simulink model "SWC_TCF"  (R2020a)
settings: Solver=FixedStepDiscrete  StartTime=0.0  StopTime=0.01  FixedStep=0.001  RelTol=1e-3
values from neighbouring files (symbols this model uses):
  CAL_TCF_AgTrqTubeCAy_af32 = 0.0    [SWC_TCF_DataDictionary.sldd]
  CAL_TCF_flgUsePlossCompa_b = 0.0    [SWC_TCF_DataDictionary.sldd]
  CAL_TCF_HiSpdDirStop_f32 = 0.0    [SWC_TCF_DataDictionary.sldd]
  CAL_TCF_HiTrqDirStop_f32 = 0.0    [SWC_TCF_DataDictionary.sldd]
  CAL_TCF_IsCutOffFrq_f32 = 0.0    [SWC_TCF_DataDictionary.sldd]
  CAL_TCF_IsPwrLosCAx_af32 = 0.0    [SWC_TCF_DataDictionary.sldd]
  CAL_TCF_LdSubLqCAzGen_af32 = 0.0    [SWC_TCF_DataDictionary.sldd]
  CAL_TCF_LdSubLqCAzMot_af32 = 0.0    [SWC_TCF_DataDictionary.sldd]
  CAL_TCF_LdSubLqIdCAx_af32 = 0.0    [SWC_TCF_DataDictionary.sldd]
  CAL_TCF_LdSubLqIqCAy_af32 = 0.0    [SWC_TCF_DataDictionary.sldd]
  CAL_TCF_LoSpdDirStop_f32 = 0.0    [SWC_TCF_DataDictionary.sldd]
  CAL_TCF_LoTrqDirStop_f32 = 0.0    [SWC_TCF_DataDictionary.sldd]
  CAL_TCF_MotorPole_u8 = 0.0    [SWC_TCF_DataDictionary.sldd]
  CAL_TCF_NPwrLosCAy_af32 = 0.0    [SWC_TCF_DataDictionary.sldd]
  CAL_TCF_Psi_f32 = 0.0    [SWC_TCF_DataDictionary.sldd]
  CAL_TCF_PwrCompaElectCAz_af32 = 0.0    [SWC_TCF_DataDictionary.sldd]
  CAL_TCF_PwrCompaIsCAy_af32 = 0.0    [SWC_TCF_DataDictionary.sldd]
  CAL_TCF_PwrCompaSpdCAx_af32 = 0.0    [SWC_TCF_DataDictionary.sldd]
  CAL_TCF_PwrInputCutOffFrq_f32 = 0.0    [SWC_TCF_DataDictionary.sldd]
  CAL_TCF_PwrLossCAz_af32 = 0.0    [SWC_TCF_DataDictionary.sldd]
  CAL_TCF_PwrTrqCalcSpdThrH_f32 = 0.0    [SWC_TCF_DataDictionary.sldd]
  CAL_TCF_PwrTrqCalcSpdThrL_f32 = 0.0    [SWC_TCF_DataDictionary.sldd]
  CAL_TCF_PwrTrqTubeCAy_af32 = 0.0    [SWC_TCF_DataDictionary.sldd]
  CAL_TCF_SpeedCtlMode_u8 = 0.0    [SWC_TCF_DataDictionary.sldd]
  CAL_TCF_TempStrMax_f32 = 0.0    [SWC_TCF_DataDictionary.sldd]
  CAL_TCF_TempStrMin_f32 = 0.0    [SWC_TCF_DataDictionary.sldd]
  CAL_TCF_TempStrPlossFact_f32 = 0.0    [SWC_TCF_DataDictionary.sldd]
  CAL_TCF_TrqCalcMonCountTrh_s16 = 0.0    [SWC_TCF_DataDictionary.sldd]
  CAL_TCF_TrqCalcMonDebTrh_s16 = 0.0    [SWC_TCF_DataDictionary.sldd]
  CAL_TCF_TrqCalcMonErrRst_b = 0.0    [SWC_TCF_DataDictionary.sldd]
  CAL_TCF_TrqMechCutOffFrq_f32 = 0.0    [SWC_TCF_DataDictionary.sldd]
  CAL_TCF_TrqTubeNCAx_af32 = 0.0    [SWC_TCF_DataDictionary.sldd]
  GLB_TCF_BwELect_u8 = 0.0    [SWC_TCF_DataDictionary.sldd]
  GLB_TCF_BwGene_u8 = 0.0    [SWC_TCF_DataDictionary.sldd]
  GLB_TCF_CircAge_f32 = 0.0    [SWC_TCF_DataDictionary.sldd]
  GLB_TCF_DigtValue_u16 = 0.0    [SWC_TCF_DataDictionary.sldd]
  GLB_TCF_FwELect_u8 = 0.0    [SWC_TCF_DataDictionary.sldd]
  GLB_TCF_FwGene_u8 = 0.0    [SWC_TCF_DataDictionary.sldd]
  GLB_TCF_MotorBw_u8 = 0.0    [SWC_TCF_DataDictionary.sldd]
  GLB_TCF_MotorFw_u8 = 0.0    [SWC_TCF_DataDictionary.sldd]
  GLB_TCF_MotorStop_u8 = 0.0    [SWC_TCF_DataDictionary.sldd]
  GLB_TCF_NegvTrq_u8 = 0.0    [SWC_TCF_DataDictionary.sldd]
  GLB_TCF_PosvTrq_u8 = 0.0    [SWC_TCF_DataDictionary.sldd]
  GLB_TCF_ZeroTrq_u8 = 0.0    [SWC_TCF_DataDictionary.sldd]
  PRV_CalFltFrq_1ms = 0.0    [SWC_TCF_DataDictionary.sldd]
  PRV_IsCalFltFrq_1ms = 0.0    [SWC_TCF_DataDictionary.sldd]
  Tbl_cos_table = 0.0    [SWC_TCF_DataDictionary.sldd]
  Tbl_sin_table = 0.0    [SWC_TCF_DataDictionary.sldd]
  TCF_PwrCompaGenCAz_af32 = 0.0    [SWC_TCF_DataDictionary.sldd]
undefined symbols (not defined in the file or in its folder): CAL_TOM_AgTrqFltTs_f32, CAL_TOM_PwrTrqFltTs_f32
libraries: simulink x9
(part 1 of 2)
settings Model: DataDictionary=SWC_TCF_DataDictionary.sldd  EnableAccessToBaseWorkspace=off  Creator=dongliyuan  LastModifiedBy=zhangjunren
settings DataIOCC: SaveFormat=StructureWithTime
settings OptimizationCC: DefaultParameterBehavior=Inlined  DefaultUnderspecifiedDataType=single  EnhancedBackFolding=on  PassReuseOutputArgsAs=Individual arguments  ZeroExternalMemoryAtStartup=off  ZeroInternalMemoryAtStartup=off  OptimizeBlockOrder=speed  DifferentSizesBufferReuse=on  OptimizationCustomize=off  EfficientTunableParamExpr=on
settings DebuggingCC: SignalInfNanChecking=warning  ParameterPrecisionLossMsg=none  ParameterTunabilityLossMsg=error  UnnecessaryDatatypeConvMsg=warning  VectorMatrixConversionMsg=warning  StrictBusMsg=WarnOnBusTreatedAsVector  NonBusSignalsTreatedAsBus=warning
settings ModelReferenceCC: ModelReferenceNumInstancesAllowed=Single
settings SFSimCC: MATLABDynamicMemAlloc=off
settings RTWCC: SystemTargetFile=ert.tlc  GenCodeOnly=on  TemplateMakefile=ert_default_tmf
settings RTWCC: CustomSourceCode=|
  | #include "set_get_data.h"
  | #include "L2Sample_FS.h"
settings CodeAppCC: ForceParamTrailComments=on  IgnoreCustomStorageClasses=off  OperatorAnnotations=on  SimulinkDataObjDesc=on  SFDataObjDesc=on  InsertBlockDesc=on
settings ERTTargetCC: TargetLangStandard=C99 (ISO)  UtilityFuncGeneration=Shared location  IncludeMdlTerminateFcn=off  SupportNonFinite=off  SupportComplex=off  GenerateASAP2=on  InlinedParameterPlacement=NonHierarchical  ERTCustomFileTemplate=example_file_process.tlc  EnableUserReplacementTypes=on

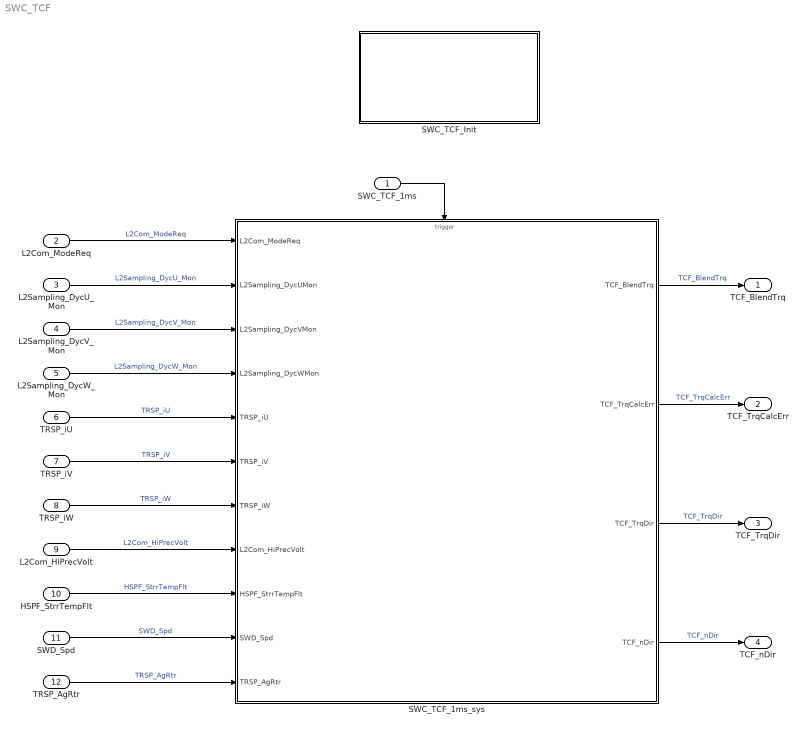
== system SWC_TCF ==
  SWC_TCF_1ms : Inport  SampleTime=0.001  OutputFunctionCall=on
  L2Com_ModeReq : Inport  Port=2  OutDataTypeStr=uint8  PortDimensions=1
  L2Sampling_DycU_Mon : Inport  Port=3  OutDataTypeStr=single  PortDimensions=1
  L2Sampling_DycV_Mon : Inport  Port=4  OutDataTypeStr=single  PortDimensions=1
  L2Sampling_DycW_Mon : Inport  Port=5  OutDataTypeStr=single  PortDimensions=1
  TRSP_iU : Inport  Port=6  OutDataTypeStr=single  PortDimensions=1
  TRSP_iV : Inport  Port=7  OutDataTypeStr=single  PortDimensions=1
  TRSP_iW : Inport  Port=8  OutDataTypeStr=single  PortDimensions=1
  L2Com_HiPrecVolt : Inport  Port=9  OutDataTypeStr=single  PortDimensions=1
  HSPF_StrrTempFlt : Inport  Port=10
  SWD_Spd : Inport  Port=11
  TRSP_AgRtr : Inport  Port=12
  SWC_TCF_1ms_sys : Subsystem
  SWC_TCF_Init : Subsystem
  TCF_BlendTrq : Outport
  TCF_TrqCalcErr : Outport  Port=2
  TCF_TrqDir : Outport  Port=3
  TCF_nDir : Outport  Port=4
  wires:
  L2Sampling_DycU_Mon/1 -> SWC_TCF_1ms_sys/2(L2Sampling_DycUMon)  "L2Sampling_DycU_Mon"
  L2Sampling_DycV_Mon/1 -> SWC_TCF_1ms_sys/3(L2Sampling_DycVMon)  "L2Sampling_DycV_Mon"
  L2Sampling_DycW_Mon/1 -> SWC_TCF_1ms_sys/4(L2Sampling_DycWMon)  "L2Sampling_DycW_Mon"
  L2Com_HiPrecVolt/1 -> SWC_TCF_1ms_sys/8(L2Com_HiPrecVolt)  "L2Com_HiPrecVolt"
  L2Com_ModeReq/1 -> SWC_TCF_1ms_sys/1(L2Com_ModeReq)  "L2Com_ModeReq"
  SWC_TCF_1ms/1 -> SWC_TCF_1ms_sys/Trigger
  HSPF_StrrTempFlt/1 -> SWC_TCF_1ms_sys/9(HSPF_StrrTempFlt)  "HSPF_StrrTempFlt"
  SWD_Spd/1 -> SWC_TCF_1ms_sys/10(SWD_Spd)  "SWD_Spd"
  TRSP_AgRtr/1 -> SWC_TCF_1ms_sys/11(TRSP_AgRtr)  "TRSP_AgRtr"
  TRSP_iU/1 -> SWC_TCF_1ms_sys/5(TRSP_iU)  "TRSP_iU"
  TRSP_iV/1 -> SWC_TCF_1ms_sys/6(TRSP_iV)  "TRSP_iV"
  TRSP_iW/1 -> SWC_TCF_1ms_sys/7(TRSP_iW)  "TRSP_iW"
  SWC_TCF_1ms_sys/1(TCF_BlendTrq) -> TCF_BlendTrq/1  "TCF_BlendTrq"
  SWC_TCF_1ms_sys/2(TCF_TrqCalcErr) -> TCF_TrqCalcErr/1  "TCF_TrqCalcErr"
  SWC_TCF_1ms_sys/3(TCF_TrqDir) -> TCF_TrqDir/1  "TCF_TrqDir"
  SWC_TCF_1ms_sys/4(TCF_nDir) -> TCF_nDir/1  "TCF_nDir"

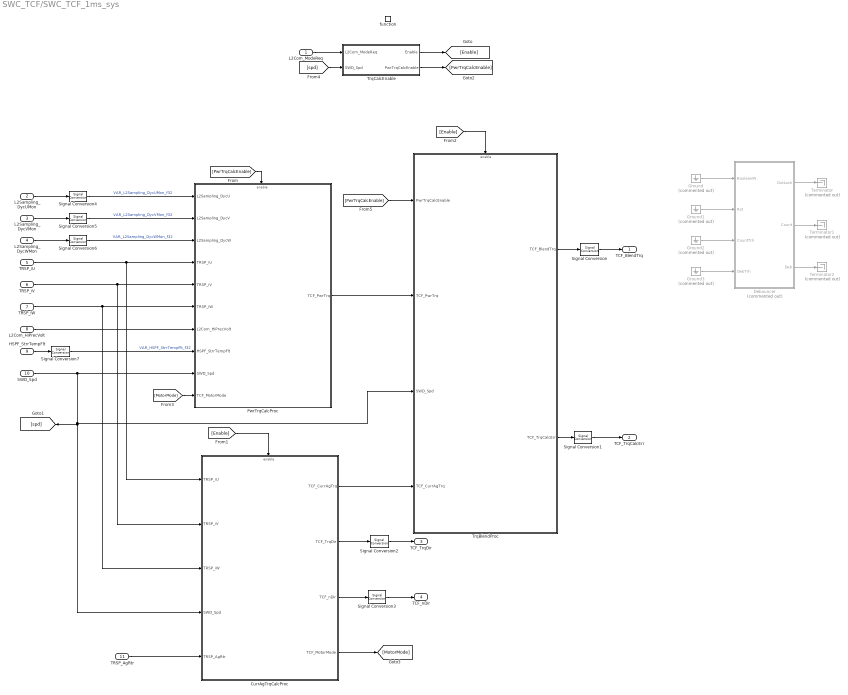
== system SWC_TCF/SWC_TCF_1ms_sys ==
  L2Com_ModeReq : Inport
  L2Sampling_DycUMon : Inport  Port=2
  L2Sampling_DycVMon : Inport  Port=3
  L2Sampling_DycWMon : Inport  Port=4
  TRSP_iU : Inport  Port=5
  TRSP_iV : Inport  Port=6
  TRSP_iW : Inport  Port=7
  L2Com_HiPrecVolt : Inport  Port=8
  HSPF_StrrTempFlt : Inport  Port=9
  SWD_Spd : Inport  Port=10
  TRSP_AgRtr : Inport  Port=11
  function : TriggerPort  TriggerType=function-call  VariantControl=(inherit)  SampleTimeType=periodic  SampleTime=-1
  CurrAgTrqCalcProc : Subsystem
  Debouncer : Subsystem  Commented=on  TreatAsAtomicUnit=on
  Ground{,1..3} (4 alike) : Ground  Commented=on
  PwrTrqCalcProc : Subsystem
  Signal Conversion{,1..7} (8 alike) : SignalConversion  OverrideOpt=off
  Terminator : Terminator  Commented=on
  Terminator1 : Terminator  Commented=on
  Terminator2 : Terminator  Commented=on
  TrqBlendProc : Subsystem
  TrqCalcEnable : Subsystem  TreatAsAtomicUnit=on
  TCF_BlendTrq : Outport
  TCF_TrqCalcErr : Outport  Port=2
  TCF_TrqDir : Outport  Port=3
  TCF_nDir : Outport  Port=4
  wires:
  CurrAgTrqCalcProc/2(TCF_TrqDir) -> Signal Conversion2/1
  TRSP_iU/1 -> PwrTrqCalcProc/4(TRSP_iU), CurrAgTrqCalcProc/1(TRSP_iU)
  TRSP_AgRtr/1 -> CurrAgTrqCalcProc/5(TRSP_AgRtr)
  TRSP_iW/1 -> PwrTrqCalcProc/6(TRSP_iW), CurrAgTrqCalcProc/3(TRSP_iW)
  HSPF_StrrTempFlt/1 -> Signal Conversion7/1
  L2Sampling_DycUMon/1 -> Signal Conversion4/1
  CurrAgTrqCalcProc/3(TCF_nDir) -> Signal Conversion3/1
  L2Com_HiPrecVolt/1 -> PwrTrqCalcProc/7(L2Com_HiPrecVolt)
  TrqBlendProc/1(TCF_BlendTrq) -> Signal Conversion/1
  TrqBlendProc/2(TCF_TrqCalcErr) -> Signal Conversion1/1
  CurrAgTrqCalcProc/1(TCF_CurrAgTrq) -> TrqBlendProc/4(TCF_CurrAgTrq)
  TRSP_iV/1 -> PwrTrqCalcProc/5(TRSP_iV), CurrAgTrqCalcProc/2(TRSP_iV)
  SWD_Spd/1 -> PwrTrqCalcProc/9(SWD_Spd), [spd], CurrAgTrqCalcProc/4(SWD_Spd), TrqBlendProc/3(SWD_Spd)
  L2Sampling_DycVMon/1 -> Signal Conversion5/1
  L2Sampling_DycWMon/1 -> Signal Conversion6/1
  [PwrTrqCalcEnable] -> PwrTrqCalcProc/Enable
  [Enable] -> CurrAgTrqCalcProc/Enable
  [Enable] -> TrqBlendProc/Enable
  Signal Conversion/1 -> TCF_BlendTrq/1
  Signal Conversion1/1 -> TCF_TrqCalcErr/1
  Signal Conversion2/1 -> TCF_TrqDir/1
  Signal Conversion3/1 -> TCF_nDir/1
  Ground/1 -> Debouncer/1(BooleanIN)
  Ground1/1 -> Debouncer/2(Rst)
  Ground2/1 -> Debouncer/3(CountTrh)
  Ground3/1 -> Debouncer/4(DebTrh)
  Debouncer/1(OutLock) -> Terminator/1
  Debouncer/2(Count) -> Terminator1/1
  Debouncer/3(Deb) -> Terminator2/1
  L2Com_ModeReq/1 -> TrqCalcEnable/1(L2Com_ModeReq)
  TrqCalcEnable/1(Enable) -> [Enable]
  Signal Conversion4/1 -> PwrTrqCalcProc/1(L2Sampling_DycU)  "VAR_L2Sampling_DycUMon_f32"
  Signal Conversion5/1 -> PwrTrqCalcProc/2(L2Sampling_DycV)  "VAR_L2Sampling_DycVMon_f32"
  Signal Conversion6/1 -> PwrTrqCalcProc/3(L2Sampling_DycW)  "VAR_L2Sampling_DycWMon_f32"
  Signal Conversion7/1 -> PwrTrqCalcProc/8(HSPF_StrrTempFlt)  "VAR_HSPF_StrrTempFlt_f32"
  [MotorMode] -> PwrTrqCalcProc/10(TCF_MotorMode)
  CurrAgTrqCalcProc/4(TCF_MotorMode) -> [MotorMode]
  [spd] -> TrqCalcEnable/2(SWD_Spd)
  TrqCalcEnable/2(PwrTrqCalcEnable) -> [PwrTrqCalcEnable]
  [PwrTrqCalcEnable] -> TrqBlendProc/1(PwrTrqCalcEnable)
  PwrTrqCalcProc/1(TCF_PwrTrq) -> TrqBlendProc/2(TCF_PwrTrq)

== system SWC_TCF/SWC_TCF_Init ==
  Event Listener : EventListener  EventName=reset

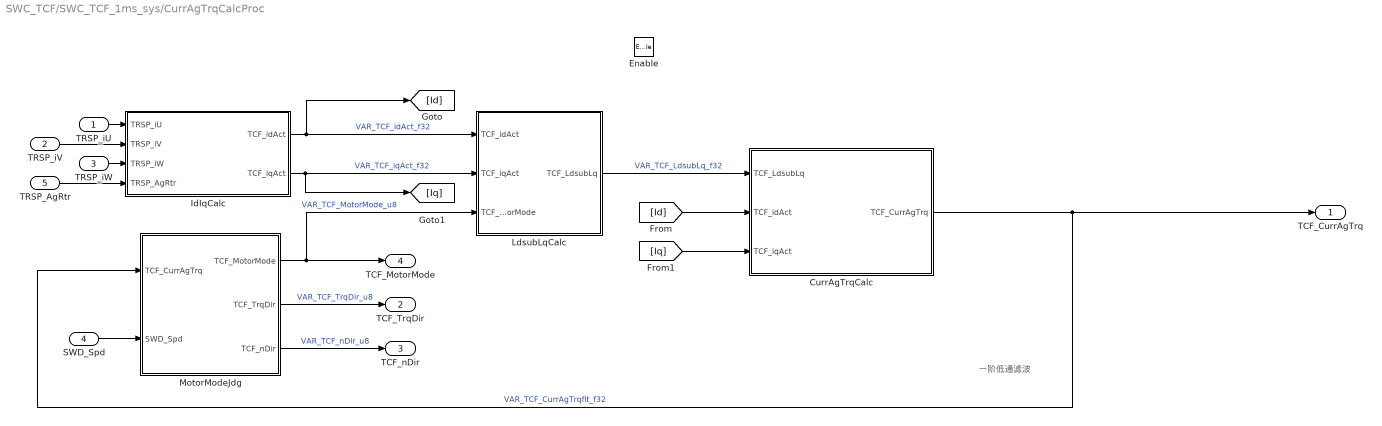
== system SWC_TCF/SWC_TCF_1ms_sys/CurrAgTrqCalcProc ==
  note: 一阶低通滤波
  TRSP_iU : Inport
  TRSP_iV : Inport  Port=2
  TRSP_iW : Inport  Port=3
  SWD_Spd : Inport  Port=4
  TRSP_AgRtr : Inport  Port=5
  Enable : EnablePort
  CurrAgTrqCalc : Subsystem  TreatAsAtomicUnit=on
      settings: RTWSystemCode=Nonreusable function
  IdIqCalc : Subsystem  TreatAsAtomicUnit=on
      settings: RTWSystemCode=Nonreusable function
  LdsubLqCalc : Subsystem  TreatAsAtomicUnit=on
      settings: RTWSystemCode=Nonreusable function
  MotorModeJdg : Subsystem  TreatAsAtomicUnit=on
      settings: RTWSystemCode=Nonreusable function
  TCF_CurrAgTrq : Outport  VectorParamsAs1DForOutWhenUnconnected=off
  TCF_TrqDir : Outport  Port=2  VectorParamsAs1DForOutWhenUnconnected=off
  TCF_nDir : Outport  Port=3  VectorParamsAs1DForOutWhenUnconnected=off
  TCF_MotorMode : Outport  Port=4
  wires:
  IdIqCalc/1(TCF_idAct) -> [Id], LdsubLqCalc/1(TCF_idAct)  "VAR_TCF_idAct_f32"
  IdIqCalc/2(TCF_iqAct) -> [Iq], LdsubLqCalc/2(TCF_iqAct)  "VAR_TCF_iqAct_f32"
  MotorModeJdg/1(TCF_MotorMode) -> LdsubLqCalc/3(TCF_MotorMode), TCF_MotorMode/1  "VAR_TCF_MotorMode_u8"
  SWD_Spd/1 -> MotorModeJdg/2(SWD_Spd)
  TRSP_iU/1 -> IdIqCalc/1(TRSP_iU)
  TRSP_iV/1 -> IdIqCalc/2(TRSP_iV)
  TRSP_iW/1 -> IdIqCalc/3(TRSP_iW)
  TRSP_AgRtr/1 -> IdIqCalc/4(TRSP_AgRtr)
  CurrAgTrqCalc/1(TCF_CurrAgTrq) -> MotorModeJdg/1(TCF_CurrAgTrq), TCF_CurrAgTrq/1  "VAR_TCF_CurrAgTrqflt_f32"
  LdsubLqCalc/1(TCF_LdsubLq) -> CurrAgTrqCalc/1(TCF_LdsubLq)  "VAR_TCF_LdsubLq_f32"
  [Id] -> CurrAgTrqCalc/2(TCF_idAct)
  [Iq] -> CurrAgTrqCalc/3(TCF_iqAct)
  MotorModeJdg/3(TCF_nDir) -> TCF_nDir/1  "VAR_TCF_nDir_u8"
  MotorModeJdg/2(TCF_TrqDir) -> TCF_TrqDir/1  "VAR_TCF_TrqDir_u8"

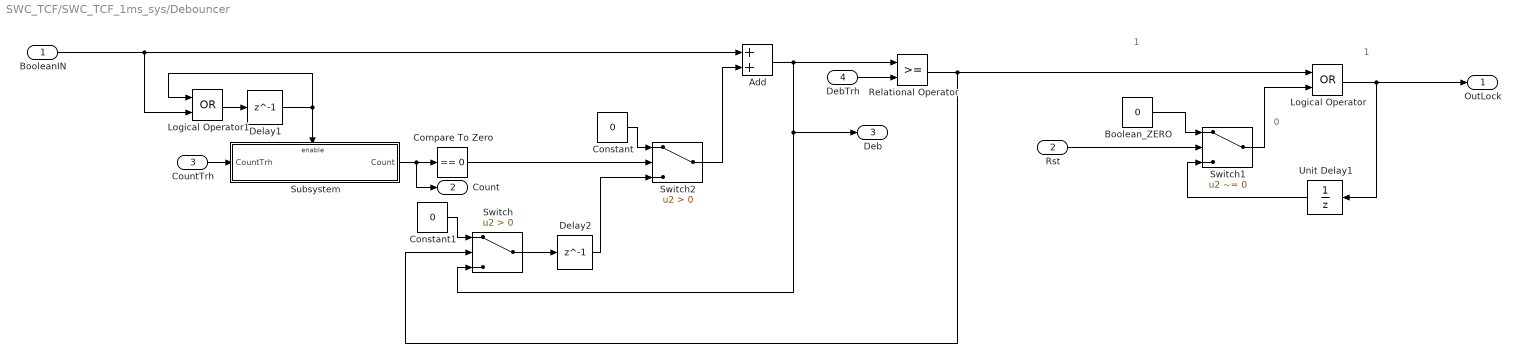
== system SWC_TCF/SWC_TCF_1ms_sys/Debouncer ==
  note: 0
  note: 1
  note: 1
  BooleanIN : Inport  OutDataTypeStr=boolean
  Rst : Inport  Port=2  OutDataTypeStr=boolean
  CountTrh : Inport  Port=3  OutDataTypeStr=int16
  DebTrh : Inport  Port=4  OutDataTypeStr=int16
  Add : Sum
  Boolean_ZERO : Constant  Value=0  OutDataTypeStr=boolean
  Compare To Zero : simulink/Logic and Bit Operations/Compare To Zero  relop===  OutDataTypeStr=boolean
  Constant : Constant  Value=0  OutDataTypeStr=int16
  Constant1 : Constant  Value=0  OutDataTypeStr=int16
  Delay1 : Delay  DelayLength=1
  Delay2 : Delay  DelayLength=1
  Logical Operator : Logic  Operator=OR  AllPortsSameDT=off  OutDataTypeStr=boolean
  Logical Operator1 : Logic  Operator=OR  AllPortsSameDT=off  OutDataTypeStr=boolean
  Relational Operator : RelationalOperator  OutDataTypeStr=boolean  RndMeth=Simplest
  Subsystem : Subsystem
  Switch : Switch  Criteria=u2 > Threshold
  Switch1 : Switch  Criteria=u2 ~= 0
  Switch2 : Switch  Criteria=u2 > Threshold
  Unit Delay1 : UnitDelay  SampleTime=-1  HasFrameUpgradeWarning=on
  OutLock : Outport  OutDataTypeStr=boolean  VectorParamsAs1DForOutWhenUnconnected=off
  Count : Outport  Port=2
  Deb : Outport  Port=3
  wires:
  Constant1/1 -> Switch/1
  Switch/1 -> Delay2/1
  DebTrh/1 -> Relational Operator/2
  Relational Operator/1 -> Logical Operator/1, Switch/2
  BooleanIN/1 -> Add/1, Logical Operator1/2
  Unit Delay1/1 -> Switch1/3
  Switch1/1 -> Logical Operator/2
  Rst/1 -> Switch1/2
  Boolean_ZERO/1 -> Switch1/1
  Logical Operator/1 -> Unit Delay1/1, OutLock/1
  Subsystem/1(Count) -> Count/1, Compare To Zero/1
  Compare To Zero/1 -> Switch2/2
  Constant/1 -> Switch2/1
  Switch2/1 -> Add/2
  Delay1/1 -> Logical Operator1/1, Subsystem/Enable
  Logical Operator1/1 -> Delay1/1
  CountTrh/1 -> Subsystem/1(CountTrh)
  Add/1 -> Deb/1, Switch/3, Relational Operator/1
  Delay2/1 -> Switch2/3

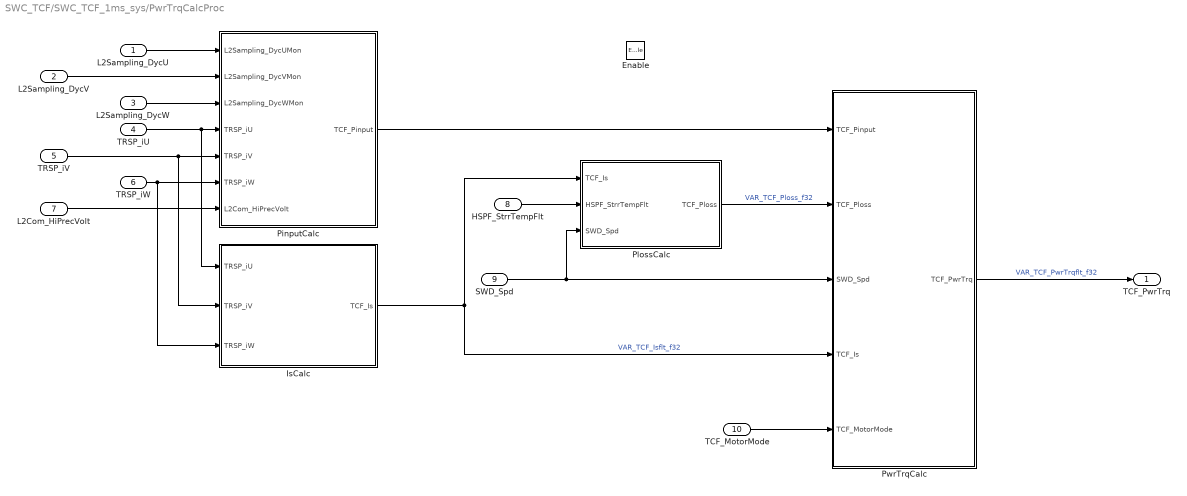
== system SWC_TCF/SWC_TCF_1ms_sys/PwrTrqCalcProc ==
  L2Sampling_DycU : Inport
  L2Sampling_DycV : Inport  Port=2
  L2Sampling_DycW : Inport  Port=3
  TRSP_iU : Inport  Port=4
  TRSP_iV : Inport  Port=5
  TRSP_iW : Inport  Port=6
  L2Com_HiPrecVolt : Inport  Port=7
  HSPF_StrrTempFlt : Inport  Port=8
  SWD_Spd : Inport  Port=9
  TCF_MotorMode : Inport  Port=10
  Enable : EnablePort
  IsCalc : Subsystem  TreatAsAtomicUnit=on
      settings: RTWSystemCode=Nonreusable function
  PinputCalc : Subsystem  TreatAsAtomicUnit=on
      settings: RTWSystemCode=Nonreusable function
  PlossCalc : Subsystem  TreatAsAtomicUnit=on
      settings: RTWSystemCode=Nonreusable function
  PwrTrqCalc : Subsystem  TreatAsAtomicUnit=on
      settings: RTWSystemCode=Nonreusable function
  TCF_PwrTrq : Outport  VectorParamsAs1DForOutWhenUnconnected=off
  wires:
  TRSP_iV/1 -> IsCalc/2(TRSP_iV), PinputCalc/5(TRSP_iV)
  TRSP_iW/1 -> IsCalc/3(TRSP_iW), PinputCalc/6(TRSP_iW)
  L2Sampling_DycU/1 -> PinputCalc/1(L2Sampling_DycUMon)
  L2Sampling_DycW/1 -> PinputCalc/3(L2Sampling_DycWMon)
  L2Com_HiPrecVolt/1 -> PinputCalc/7(L2Com_HiPrecVolt)
  L2Sampling_DycV/1 -> PinputCalc/2(L2Sampling_DycVMon)
  TRSP_iU/1 -> IsCalc/1(TRSP_iU), PinputCalc/4(TRSP_iU)
  PlossCalc/1(TCF_Ploss) -> PwrTrqCalc/2(TCF_Ploss)  "VAR_TCF_Ploss_f32"
  PinputCalc/1(TCF_Pinput) -> PwrTrqCalc/1(TCF_Pinput)
  HSPF_StrrTempFlt/1 -> PlossCalc/2(HSPF_StrrTempFlt)
  IsCalc/1(TCF_Is) -> PwrTrqCalc/4(TCF_Is), PlossCalc/1(TCF_Is)  "VAR_TCF_Isflt_f32"
  PwrTrqCalc/1(TCF_PwrTrq) -> TCF_PwrTrq/1  "VAR_TCF_PwrTrqflt_f32"
  TCF_MotorMode/1 -> PwrTrqCalc/5(TCF_MotorMode)
  SWD_Spd/1 -> PlossCalc/3(SWD_Spd), PwrTrqCalc/3(SWD_Spd)

== system SWC_TCF/SWC_TCF_1ms_sys/TrqBlendProc ==
  PwrTrqCalcEnable : Inport
  TCF_PwrTrq : Inport  Port=2
  SWD_Spd : Inport  Port=3
  TCF_CurrAgTrq : Inport  Port=4
  Enable : EnablePort
  CAL_TOM_HiTrqMonDebTrh_s4 : Constant  Value=CAL_TCF_TrqCalcMonDebTrh_s16  OutDataTypeStr=int16
  CAL_TOM_HiTrqMonDebTrh_s5 : Constant  Value=CAL_TCF_TrqCalcMonCountTrh_s16  OutDataTypeStr=int16
  CAL_TOM_TrqMonErrRst_b2 : Constant  Value=CAL_TCF_TrqCalcMonErrRst_b  OutDataTypeStr=boolean
  Debouncer : Subsystem  TreatAsAtomicUnit=on
  TrqBlend : Subsystem  TreatAsAtomicUnit=on
      settings: RTWSystemCode=Nonreusable function
  TrqTube : Subsystem  TreatAsAtomicUnit=on
      settings: RTWSystemCode=Nonreusable function
  TCF_BlendTrq : Outport  VectorParamsAs1DForOutWhenUnconnected=off
  TCF_TrqCalcErr : Outport  Port=2  VectorParamsAs1DForOutWhenUnconnected=off
  wires:
  TCF_PwrTrq/1 -> TrqTube/2(TCF_PwrTrq)
  TCF_CurrAgTrq/1 -> TrqTube/4(TCF_CurrAgTrq)
  TrqBlend/1(TCF_BlendTrq) -> TCF_BlendTrq/1  "VAR_TCF_BlendTrq_f32"
  TrqTube/1(TCF_PwrTrq_TubeH) -> TrqBlend/1(TCF_PwrTrq_TubeH)  "VAR_TCF_PwrTrqTubeH1_f32"
  TrqTube/2(TCF_PwrTrq_TubeL) -> TrqBlend/2(TCF_PwrTrq_TubeL)  "VAR_TCF_PwrTrqTubeL1_f32"
  TrqTube/3(TCF_CurrAgTrq_TubeH) -> TrqBlend/3(TCF_CurrAgTrq_TubeH)  "VAR_TCF_CurrAgTrqTubeH1_f32"
  TrqTube/4(TCF_CurrAgTrq_TubeL) -> TrqBlend/4(TCF_CurrAgTrq_TubeL)  "VAR_TCF_CurrAgTrqTubeL1_f32"
  Debouncer/1(OutLock) -> TCF_TrqCalcErr/1  "VAR_TCF_TrqCalcErr_b"
  SWD_Spd/1 -> TrqTube/3(SWD_Spd)
  CAL_TOM_HiTrqMonDebTrh_s4/1 -> Debouncer/4(DebTrh)
  TrqBlend/2(TCF_TrqCalcMonRslt) -> Debouncer/1(BooleanIN)  "VAR_TCF_TrqCalcMonRslt_b"
  CAL_TOM_TrqMonErrRst_b2/1 -> Debouncer/2(Rst)
  CAL_TOM_HiTrqMonDebTrh_s5/1 -> Debouncer/3(CountTrh)
  PwrTrqCalcEnable/1 -> TrqTube/1(PwrTrqCalcEnable)

== system SWC_TCF/SWC_TCF_1ms_sys/TrqCalcEnable ==
  L2Com_ModeReq : Inport
  SWD_Spd : Inport  Port=2
  Abs : Abs
  CAL_TOM_SpeedCtlMode_u8 : Constant  Value=CAL_TCF_SpeedCtlMode_u8  OutDataTypeStr=uint8
  Logical Operator : Logic  AllPortsSameDT=off  OutDataTypeStr=boolean
  Relational Operator2 : RelationalOperator  Operator=~=  OutDataTypeStr=boolean  RndMeth=Simplest
  Relay : Relay  OnSwitchValue=CAL_TCF_PwrTrqCalcSpdThrH_f32  OffSwitchValue=CAL_TCF_PwrTrqCalcSpdThrL_f32
  Enable : Outport
  PwrTrqCalcEnable : Outport  Port=2
  wires:
  Relational Operator2/1 -> Logical Operator/1, Enable/1
  CAL_TOM_SpeedCtlMode_u8/1 -> Relational Operator2/2
  L2Com_ModeReq/1 -> Relational Operator2/1
  SWD_Spd/1 -> Abs/1
  Abs/1 -> Relay/1
  Logical Operator/1 -> PwrTrqCalcEnable/1
  Relay/1 -> Logical Operator/2

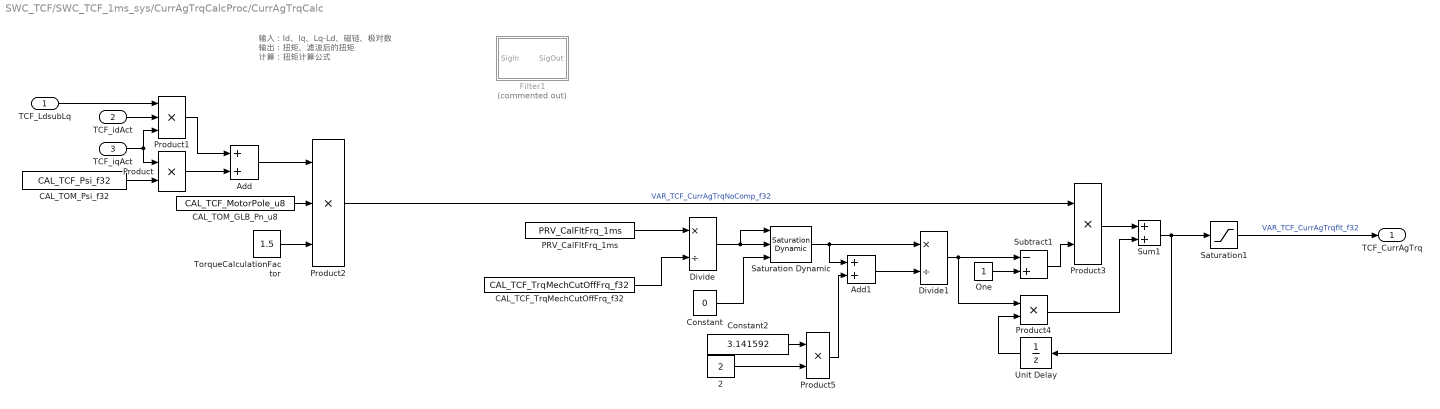
== system SWC_TCF/SWC_TCF_1ms_sys/CurrAgTrqCalcProc/CurrAgTrqCalc ==
  note: 输入：Id、Iq、Lq-Ld、磁链、极对数
      | 输出：扭矩、滤波后的扭矩
      |
      | 计算：扭矩计算公式
  TCF_LdsubLq : Inport
  TCF_idAct : Inport  Port=2
  TCF_iqAct : Inport  Port=3
  2 : Constant  Value=2  OutDataTypeStr=single
  Add : Sum
  Add1 : Sum
  CAL_TCF_TrqMechCutOffFrq_f32 : Constant  Value=CAL_TCF_TrqMechCutOffFrq_f32
  CAL_TOM_GLB_Pn_u8 : Constant  Value=CAL_TCF_MotorPole_u8  OutDataTypeStr=uint8
  CAL_TOM_Psi_f32 : Constant  Value=CAL_TCF_Psi_f32  OutDataTypeStr=single
  Constant : Constant  Value=0  OutDataTypeStr=single
  Constant2 : Constant  Value=3.141592  OutDataTypeStr=single
  Divide : Product  Inputs=*/
  Divide1 : Product  Inputs=*/
  Filter1 : Subsystem  Commented=on
  One : Constant  OutDataTypeStr=single
  PRV_CalFltFrq_1ms : Constant  Value=PRV_CalFltFrq_1ms
  Product{,3..5} (4 alike) : Product
  Product1 : Product  Inputs=3
  Product2 : Product  Inputs=3
  Saturation Dynamic : simulink/Discontinuities/Saturation Dynamic  OutMin=[]  OutMax=[]  OutDataTypeStr=Inherit: Same as second input  OutDataType=fixdt(1, 16)  OutScaling=2^-10  DoSatur=off
  Saturation1 : Saturate  UpperLimit=500  LowerLimit=-500
  Subtract1 : Sum  Inputs=-+
  Sum1 : Sum
  TorqueCalculationFactor : Constant  Value=1.5  OutDataTypeStr=single
  Unit Delay : UnitDelay  SampleTime=-1  HasFrameUpgradeWarning=on
  TCF_CurrAgTrq : Outport
  wires:
  TCF_idAct/1 -> Product1/2
  CAL_TOM_Psi_f32/1 -> Product/2
  Product1/1 -> Add/1
  TorqueCalculationFactor/1 -> Product2/3
  CAL_TOM_GLB_Pn_u8/1 -> Product2/2
  Product/1 -> Add/2
  Add/1 -> Product2/1
  TCF_LdsubLq/1 -> Product1/1
  TCF_iqAct/1 -> Product/1, Product1/3
  Constant2/1 -> Product5/1
  PRV_CalFltFrq_1ms/1 -> Divide/1
  2/1 -> Product5/2
  Saturation Dynamic/1 -> Divide1/1, Add1/1
  Constant/1 -> Saturation Dynamic/3
  One/1 -> Subtract1/2
  CAL_TCF_TrqMechCutOffFrq_f32/1 -> Divide/2
  Product3/1 -> Sum1/1
  Add1/1 -> Divide1/2
  Divide1/1 -> Product4/1, Subtract1/1
  Divide/1 -> Saturation Dynamic/1, Saturation Dynamic/2
  Subtract1/1 -> Product3/2
  Product4/1 -> Sum1/2
  Unit Delay/1 -> Product4/2
  Product5/1 -> Add1/2
  Sum1/1 -> Saturation1/1, Unit Delay/1
  Saturation1/1 -> TCF_CurrAgTrq/1  "VAR_TCF_CurrAgTrqflt_f32"
  Product2/1 -> Product3/1  "VAR_TCF_CurrAgTrqNoComp_f32"

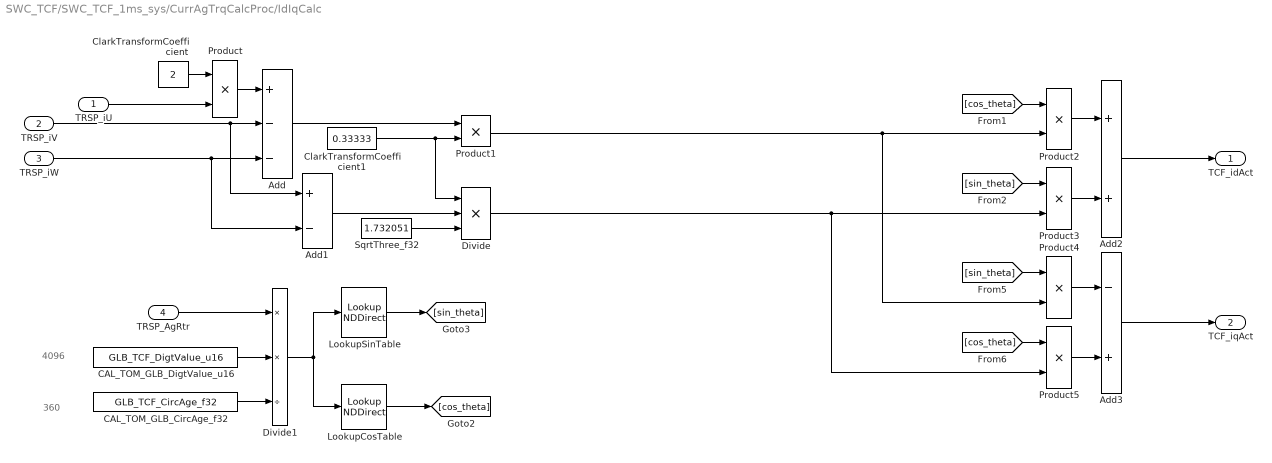
== system SWC_TCF/SWC_TCF_1ms_sys/CurrAgTrqCalcProc/IdIqCalc ==
  note: 4096
  note: 360
  TRSP_iU : Inport
  TRSP_iV : Inport  Port=2
  TRSP_iW : Inport  Port=3
  TRSP_AgRtr : Inport  Port=4
  Add : Sum  Inputs=+--
  Add1 : Sum  Inputs=+-
  Add2 : Sum
  Add3 : Sum  Inputs=-+
  CAL_TOM_GLB_CircAge_f32 : Constant  Value=GLB_TCF_CircAge_f32
  CAL_TOM_GLB_DigtValue_u16 : Constant  Value=GLB_TCF_DigtValue_u16
  ClarkTransformCoefficient : Constant  Value=2  OutDataTypeStr=single
  ClarkTransformCoefficient1 : Constant  Value=0.33333  OutDataTypeStr=single
  Divide : Product  Inputs=***
  Divide1 : Product  Inputs=**/
  LookupCosTable : LookupNDDirect  NumberOfTableDimensions=1  Table=Tbl_cos_table
  LookupSinTable : LookupNDDirect  NumberOfTableDimensions=1  Table=Tbl_sin_table
  Product{,1..5} (6 alike) : Product
  SqrtThree_f32 : Constant  Value=1.732051  OutDataTypeStr=single
  TCF_idAct : Outport  VectorParamsAs1DForOutWhenUnconnected=off
  TCF_iqAct : Outport  Port=2  VectorParamsAs1DForOutWhenUnconnected=off
  wires:
  TRSP_iW/1 -> Add1/2, Add/3
  Product/1 -> Add/1
  ClarkTransformCoefficient/1 -> Product/1
  TRSP_iV/1 -> Add1/1, Add/2
  SqrtThree_f32/1 -> Divide/3
  ClarkTransformCoefficient1/1 -> Divide/1, Product1/2
  Add1/1 -> Divide/2
  TRSP_iU/1 -> Product/2
  Add/1 -> Product1/1
  Divide1/1 -> LookupCosTable/1, LookupSinTable/1
  CAL_TOM_GLB_CircAge_f32/1 -> Divide1/3
  Product2/1 -> Add2/1
  Product4/1 -> Add3/1
  LookupCosTable/1 -> [cos_theta]
  [sin_theta] -> Product3/1
  LookupSinTable/1 -> [sin_theta]
  Product3/1 -> Add2/2
  [sin_theta] -> Product4/1
  CAL_TOM_GLB_DigtValue_u16/1 -> Divide1/2
  [cos_theta] -> Product2/1
  Product1/1 -> Product2/2, Product4/2
  [cos_theta] -> Product5/1
  Product5/1 -> Add3/2
  Divide/1 -> Product5/2, Product3/2
  TRSP_AgRtr/1 -> Divide1/1
  Add2/1 -> TCF_idAct/1
  Add3/1 -> TCF_iqAct/1

== system SWC_TCF/SWC_TCF_1ms_sys/CurrAgTrqCalcProc/LdsubLqCalc ==
  note: 后退电动
  note: 前进电动
  note: 怎么标定Ld、Lq
      |
      | 用L1层的表
  TCF_idAct : Inport
  TCF_iqAct : Inport  Port=2
  TCF_MotorMode : Inport  Port=3
  Abs : Abs
  Abs1 : Abs
  Constant : Constant  Value=GLB_TCF_FwELect_u8  OutDataTypeStr=uint8
  Constant1 : Constant  Value=GLB_TCF_BwELect_u8  OutDataTypeStr=uint8
  LdSubLqGen_L2 : Lookup_n-D  BreakpointsForDimension1=CAL_TCF_LdSubLqIdCAx_af32  BreakpointsForDimension2=CAL_TCF_LdSubLqIqCAy_af32  Table=CAL_TCF_LdSubLqCAzGen_af32  ExtrapMethod=Clip  InternalRulePriority=Speed  RndMeth=Simplest  InputSameDT=on
  LdSubLqMot_L2 : Lookup_n-D  BreakpointsForDimension1=CAL_TCF_LdSubLqIdCAx_af32  BreakpointsForDimension2=CAL_TCF_LdSubLqIqCAy_af32  Table=CAL_TCF_LdSubLqCAzMot_af32  ExtrapMethod=Clip  InternalRulePriority=Speed  RndMeth=Simplest  InputSameDT=on
  Logical Operator : Logic  Operator=OR  AllPortsSameDT=off  OutDataTypeStr=boolean
  Relational Operator : RelationalOperator  Operator===  OutDataTypeStr=boolean  RndMeth=Simplest
  Relational Operator1 : RelationalOperator  Operator===  OutDataTypeStr=boolean  RndMeth=Simplest
  Switch : Switch  Criteria=u2 ~= 0
  TCF_LdsubLq : Outport
  wires:
  Constant1/1 -> Relational Operator1/2
  Constant/1 -> Relational Operator/2
  TCF_MotorMode/1 -> Relational Operator/1, Relational Operator1/1
  Relational Operator1/1 -> Logical Operator/2
  Relational Operator/1 -> Logical Operator/1
  Logical Operator/1 -> Switch/2
  TCF_idAct/1 -> Abs/1
  TCF_iqAct/1 -> Abs1/1
  LdSubLqMot_L2/1 -> Switch/1
  Switch/1 -> TCF_LdsubLq/1
  Abs1/1 -> LdSubLqGen_L2/2, LdSubLqMot_L2/2
  Abs/1 -> LdSubLqMot_L2/1, LdSubLqGen_L2/1
  LdSubLqGen_L2/1 -> Switch/3

== system SWC_TCF/SWC_TCF_1ms_sys/CurrAgTrqCalcProc/MotorModeJdg ==
  TCF_CurrAgTrq : Inport
  SWD_Spd : Inport  Port=2
  MotorMode : Subsystem
  TrqDir : Subsystem
  nDir : Subsystem
  TCF_MotorMode : Outport  VectorParamsAs1DForOutWhenUnconnected=off
  TCF_TrqDir : Outport  Port=2  VectorParamsAs1DForOutWhenUnconnected=off
  TCF_nDir : Outport  Port=3  VectorParamsAs1DForOutWhenUnconnected=off
  wires:
  MotorMode/1(TCF_MotorMod) -> TCF_MotorMode/1
  nDir/1(TCF_nDir) -> MotorMode/2(TCF_nDir), TCF_nDir/1
  TrqDir/1(TCF_TrqDir) -> TCF_TrqDir/1, MotorMode/1(TCF_TrqDir)
  TCF_CurrAgTrq/1 -> TrqDir/1(TCF_CurrAgTrqFlt)
  SWD_Spd/1 -> nDir/1(SWD_Spd)

== system SWC_TCF/SWC_TCF_1ms_sys/Debouncer/Subsystem ==
  CountTrh : Inport
  Enable : EnablePort
  Add : Sum
  Constant : Constant  OutDataTypeStr=int16
  Constant1 : Constant  Value=0  OutDataTypeStr=int16
  Delay : Delay  DelayLength=1
  Relational Operator : RelationalOperator  OutDataTypeStr=boolean  RndMeth=Simplest
  Switch : Switch  Criteria=u2 > Threshold
  Count : Outport
  wires:
  Switch/1 -> Delay/1, Count/1
  Constant/1 -> Add/1
  Relational Operator/1 -> Switch/2
  Add/1 -> Relational Operator/1, Switch/3
  Constant1/1 -> Switch/1
  CountTrh/1 -> Relational Operator/2
  Delay/1 -> Add/2

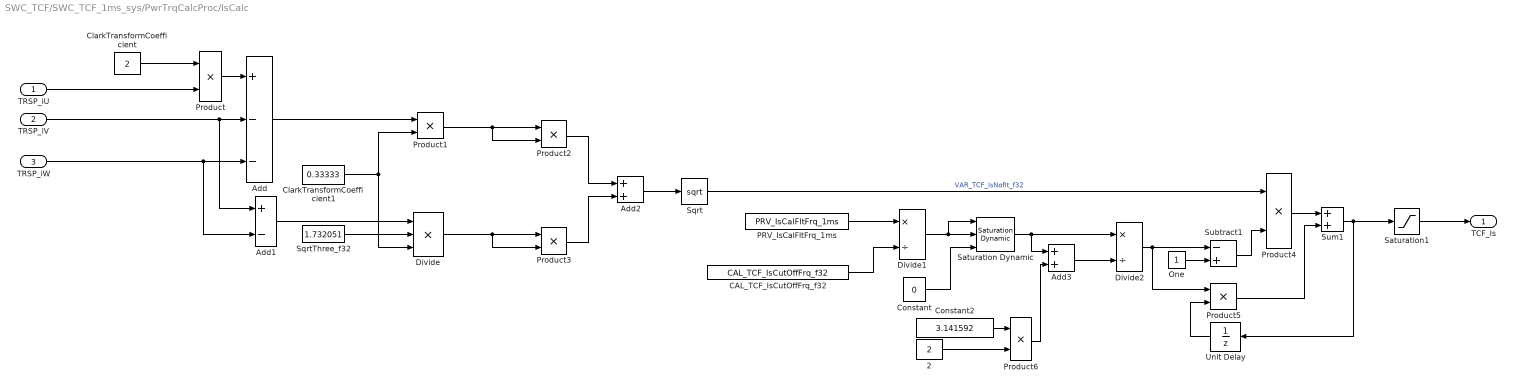
== system SWC_TCF/SWC_TCF_1ms_sys/PwrTrqCalcProc/IsCalc ==
  TRSP_iU : Inport
  TRSP_iV : Inport  Port=2
  TRSP_iW : Inport  Port=3
  2 : Constant  Value=2  OutDataTypeStr=single
  Add : Sum  Inputs=+--
  Add1 : Sum  Inputs=+-
  Add2 : Sum
  Add3 : Sum
  CAL_TCF_IsCutOffFrq_f32 : Constant  Value=CAL_TCF_IsCutOffFrq_f32
  ClarkTransformCoefficient : Constant  Value=2  OutDataTypeStr=single
  ClarkTransformCoefficient1 : Constant  Value=0.33333  OutDataTypeStr=single
  Constant : Constant  Value=0  OutDataTypeStr=single
  Constant2 : Constant  Value=3.141592  OutDataTypeStr=single
  Divide : Product  Inputs=***
  Divide1 : Product  Inputs=*/
  Divide2 : Product  Inputs=*/
  One : Constant  OutDataTypeStr=single
  PRV_IsCalFltFrq_1ms : Constant  Value=PRV_IsCalFltFrq_1ms
  Product{,1..6} (7 alike) : Product
  Saturation Dynamic : simulink/Discontinuities/Saturation Dynamic  OutMin=[]  OutMax=[]  OutDataTypeStr=Inherit: Same as second input  OutDataType=fixdt(1, 16)  OutScaling=2^-10  DoSatur=off
  Saturation1 : Saturate  UpperLimit=1000  LowerLimit=0
  Sqrt : Sqrt  SaturateOnIntegerOverflow=on
  SqrtThree_f32 : Constant  Value=1.732051  OutDataTypeStr=single
  Subtract1 : Sum  Inputs=-+
  Sum1 : Sum
  Unit Delay : UnitDelay  SampleTime=-1  HasFrameUpgradeWarning=on
  TCF_Is : Outport
  wires:
  Add/1 -> Product1/1
  SqrtThree_f32/1 -> Divide/2
  Add1/1 -> Divide/1
  ClarkTransformCoefficient/1 -> Product/1
  Product/1 -> Add/1
  TRSP_iW/1 -> Add1/2, Add/3
  TRSP_iV/1 -> Add1/1, Add/2
  ClarkTransformCoefficient1/1 -> Product1/2, Divide/3
  TRSP_iU/1 -> Product/2
  Product2/1 -> Add2/1
  Product3/1 -> Add2/2
  Add2/1 -> Sqrt/1
  Divide/1 -> Product3/2, Product3/1
  Product1/1 -> Product2/1, Product2/2
  Sum1/1 -> Unit Delay/1, Saturation1/1
  Divide1/1 -> Saturation Dynamic/1, Saturation Dynamic/2
  Product6/1 -> Add3/2
  Product5/1 -> Sum1/2
  Unit Delay/1 -> Product5/2
  One/1 -> Subtract1/2
  Sqrt/1 -> Product4/1  "VAR_TCF_IsNoflt_f32"
  Add3/1 -> Divide2/2
  Divide2/1 -> Product5/1, Subtract1/1
  Constant/1 -> Saturation Dynamic/3
  Subtract1/1 -> Product4/2
  PRV_IsCalFltFrq_1ms/1 -> Divide1/1
  Saturation Dynamic/1 -> Divide2/1, Add3/1
  Product4/1 -> Sum1/1
  2/1 -> Product6/2
  Constant2/1 -> Product6/1
  CAL_TCF_IsCutOffFrq_f32/1 -> Divide1/2
  Saturation1/1 -> TCF_Is/1

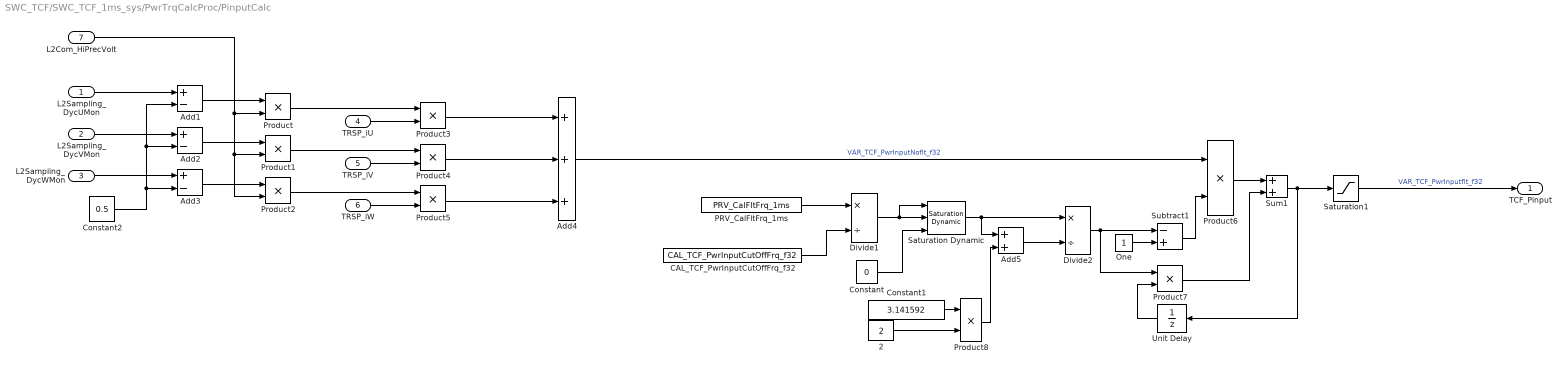
== system SWC_TCF/SWC_TCF_1ms_sys/PwrTrqCalcProc/PinputCalc ==
  L2Sampling_DycUMon : Inport
  L2Sampling_DycVMon : Inport  Port=2
  L2Sampling_DycWMon : Inport  Port=3
  TRSP_iU : Inport  Port=4
  TRSP_iV : Inport  Port=5
  TRSP_iW : Inport  Port=6
  L2Com_HiPrecVolt : Inport  Port=7
  2 : Constant  Value=2  OutDataTypeStr=single
  Add1 : Sum  Inputs=+-
  Add2 : Sum  Inputs=+-
  Add3 : Sum  Inputs=+-
  Add4 : Sum  Inputs=+++
  Add5 : Sum
  CAL_TCF_PwrInputCutOffFrq_f32 : Constant  Value=CAL_TCF_PwrInputCutOffFrq_f32
  Constant : Constant  Value=0  OutDataTypeStr=single
  Constant1 : Constant  Value=3.141592  OutDataTypeStr=single
  Constant2 : Constant  Value=0.5  OutDataTypeStr=single
  Divide1 : Product  Inputs=*/
  Divide2 : Product  Inputs=*/
  One : Constant  OutDataTypeStr=single
  PRV_CalFltFrq_1ms : Constant  Value=PRV_CalFltFrq_1ms
  Product{,1..2,6..8} (6 alike) : Product
  Product3 : Product  Inputs=**
  Product4 : Product  Inputs=**
  Product5 : Product  Inputs=**
  Saturation Dynamic : simulink/Discontinuities/Saturation Dynamic  OutMin=[]  OutMax=[]  OutDataTypeStr=Inherit: Same as second input  OutDataType=fixdt(1, 16)  OutScaling=2^-10  DoSatur=off
  Saturation1 : Saturate  UpperLimit=200000  LowerLimit=-200000
  Subtract1 : Sum  Inputs=-+
  Sum1 : Sum
  Unit Delay : UnitDelay  SampleTime=-1  HasFrameUpgradeWarning=on
  TCF_Pinput : Outport
  wires:
  Constant2/1 -> Add3/2, Add2/2, Add1/2
  Add1/1 -> Product/1
  Add2/1 -> Product1/1
  Add3/1 -> Product2/1
  L2Com_HiPrecVolt/1 -> Product2/2, Product1/2, Product/2
  L2Sampling_DycUMon/1 -> Add1/1
  L2Sampling_DycVMon/1 -> Add2/1
  L2Sampling_DycWMon/1 -> Add3/1
  Product/1 -> Product3/1
  TRSP_iV/1 -> Product4/2
  Product5/1 -> Add4/3
  Product2/1 -> Product5/1
  TRSP_iW/1 -> Product5/2
  TRSP_iU/1 -> Product3/2
  Product4/1 -> Add4/2
  Product3/1 -> Add4/1
  Product1/1 -> Product4/1
  CAL_TCF_PwrInputCutOffFrq_f32/1 -> Divide1/2
  Sum1/1 -> Saturation1/1, Unit Delay/1
  Saturation1/1 -> TCF_Pinput/1  "VAR_TCF_PwrInputflt_f32"
  Product8/1 -> Add5/2
  Add5/1 -> Divide2/2
  Saturation Dynamic/1 -> Divide2/1, Add5/1
  Product6/1 -> Sum1/1
  Constant/1 -> Saturation Dynamic/3
  Divide2/1 -> Product7/1, Subtract1/1
  One/1 -> Subtract1/2
  Unit Delay/1 -> Product7/2
  Constant1/1 -> Product8/1
  2/1 -> Product8/2
  Product7/1 -> Sum1/2
  PRV_CalFltFrq_1ms/1 -> Divide1/1
  Subtract1/1 -> Product6/2
  Divide1/1 -> Saturation Dynamic/1, Saturation Dynamic/2
  Add4/1 -> Product6/1  "VAR_TCF_PwrInputNoflt_f32"

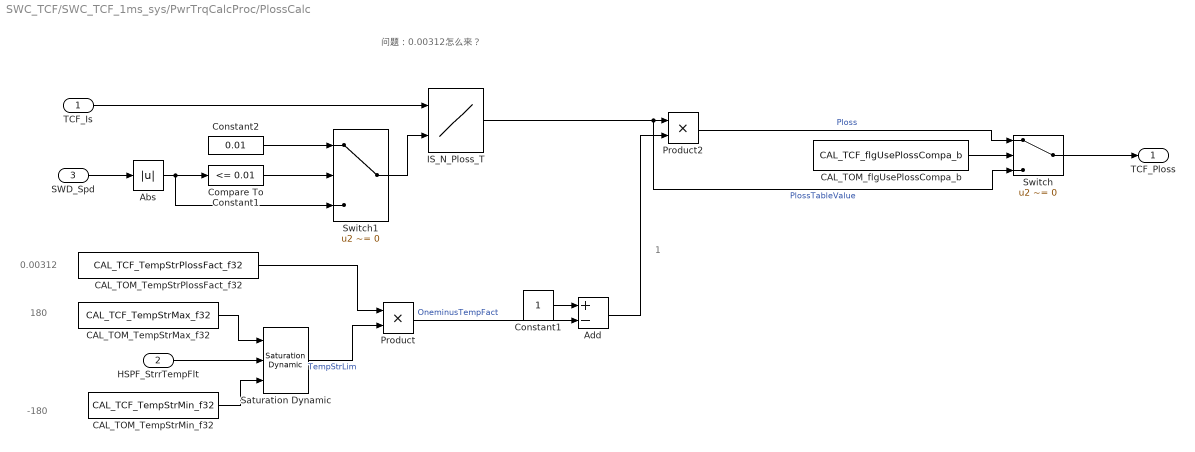
== system SWC_TCF/SWC_TCF_1ms_sys/PwrTrqCalcProc/PlossCalc ==
  note: 问题：0.00312怎么来？
  note: 1
  note: 0.00312
  note: -180
  note: 180
  TCF_Is : Inport
  HSPF_StrrTempFlt : Inport  Port=2
  SWD_Spd : Inport  Port=3
  Abs : Abs
  Add : Sum  Inputs=+-
  CAL_TOM_TempStrMax_f32 : Constant  Value=CAL_TCF_TempStrMax_f32  OutDataTypeStr=single
  CAL_TOM_TempStrMin_f32 : Constant  Value=CAL_TCF_TempStrMin_f32  OutDataTypeStr=single
  CAL_TOM_TempStrPlossFact_f32 : Constant  Value=CAL_TCF_TempStrPlossFact_f32  OutDataTypeStr=single
  CAL_TOM_flgUsePlossCompa_b : Constant  Value=CAL_TCF_flgUsePlossCompa_b  OutDataTypeStr=boolean
  Compare To Constant1 : simulink/Logic and Bit Operations/Compare To Constant  relop=<=  const=0.01  OutDataTypeStr=boolean
  Constant1 : Constant  OutDataTypeStr=single
  Constant2 : Constant  Value=0.01  OutDataTypeStr=single
  IS_N_Ploss_T : Lookup_n-D  BreakpointsForDimension1=CAL_TCF_IsPwrLosCAx_af32  BreakpointsForDimension2=CAL_TCF_NPwrLosCAy_af32  Table=CAL_TCF_PwrLossCAz_af32  InternalRulePriority=Speed  RndMeth=Simplest  InputSameDT=on
  Product : Product
  Product2 : Product
  Saturation Dynamic : simulink/Discontinuities/Saturation Dynamic  OutMin=[]  OutMax=[]  OutDataTypeStr=Inherit: Same as second input  OutDataType=fixdt(1, 16)  OutScaling=2^-10  DoSatur=off
  Switch : Switch  Criteria=u2 ~= 0
  Switch1 : Switch  Criteria=u2 ~= 0
  TCF_Ploss : Outport  VectorParamsAs1DForOutWhenUnconnected=off
  wires:
  TCF_Is/1 -> IS_N_Ploss_T/1
  SWD_Spd/1 -> Abs/1
  Product2/1 -> Switch/1  "Ploss"
  HSPF_StrrTempFlt/1 -> Saturation Dynamic/2
  CAL_TOM_TempStrMax_f32/1 -> Saturation Dynamic/1
  CAL_TOM_TempStrMin_f32/1 -> Saturation Dynamic/3
  Saturation Dynamic/1 -> Product/2  "TempStrLim"
  CAL_TOM_TempStrPlossFact_f32/1 -> Product/1
  Product/1 -> Add/2  "OneminusTempFact"
  Constant1/1 -> Add/1
  IS_N_Ploss_T/1 -> Switch/3, Product2/1  "PlossTableValue"
  Add/1 -> Product2/2
  Switch/1 -> TCF_Ploss/1
  CAL_TOM_flgUsePlossCompa_b/1 -> Switch/2
  Compare To Constant1/1 -> Switch1/2
  Abs/1 -> Switch1/3, Compare To Constant1/1
  Constant2/1 -> Switch1/1
  Switch1/1 -> IS_N_Ploss_T/2
